simulink model "ForLoop_Factorial"  (R2017b)
settings: Solver=FixedStepDiscrete  StartTime=0.0  StopTime=10.0  RelTol=1e-3
settings Model: Creator=engdo  LastModifiedBy=engdo
settings OptimizationCC: DefaultParameterBehavior=Inlined  PassReuseOutputArgsAs=Individual arguments
settings DebuggingCC: ParameterTunabilityLossMsg=error
settings SFSimCC: MATLABDynamicMemAlloc=off
settings RTWCC: SystemTargetFile=ert.tlc  GenCodeOnly=on  TemplateMakefile=ert_default_tmf  GenerateReport=on  IncludeHyperlinkInReport=on  LaunchReport=on  GenerateTraceInfo=on  GenerateTraceReport=on  GenerateTraceReportSl=on  GenerateTraceReportSf=on  GenerateTraceReportEml=on  GenerateWebview=on
settings CodeAppCC: ForceParamTrailComments=on  IgnoreCustomStorageClasses=off  OperatorAnnotations=on  SimulinkDataObjDesc=on  SFDataObjDesc=on  InsertBlockDesc=on
settings ERTTargetCC: TargetLangStandard=C99 (ISO)  GenerateSampleERTMain=on  InlinedParameterPlacement=NonHierarchical  ERTCustomFileTemplate=example_file_process.tlc  EnableUserReplacementTypes=on

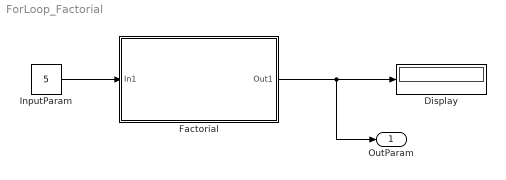
== system ForLoop_Factorial ==
  Display : Display
  Factorial : Subsystem  TreatAsAtomicUnit=on
  InputParam : Constant  Value=5
  OutParam : Outport
  wires:
  Factorial/1(Out1) -> OutParam/1, Display/1
  InputParam/1 -> Factorial/1(In1)

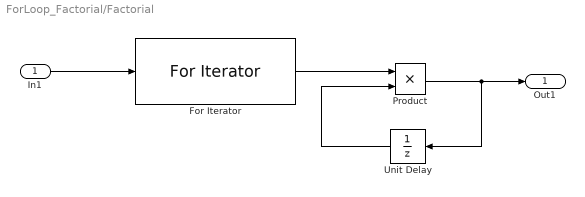
== system ForLoop_Factorial/Factorial ==
  In1 : Inport
  For Iterator : ForIterator  ResetStates=reset  IterationSource=external
  Product : Product  OutDataTypeStr=int32
  Unit Delay : UnitDelay  InitialCondition=1  SampleTime=-1
  Out1 : Outport
  wires:
  In1/1 -> For Iterator/1
  For Iterator/1 -> Product/1
  Product/1 -> Unit Delay/1, Out1/1
  Unit Delay/1 -> Product/2
